simulink model "Chaotic_synchronization_Neelabhro"  (R2019a)
settings: Solver=ode45  StartTime=0.0  StopTime=100  RelTol=1e-3  EnableMultiTasking=on
settings Model: Creator=Administrator  LastModifiedBy=ar-neelabhro.roy
settings DataIOCC: LimitDataPoints=on  SaveFormat=Array  ReturnWorkspaceOutputs=off
settings OptimizationCC: LifeSpan=inf
settings DebuggingCC: SolverPrmCheckMsg=warning  AllowSymbolicDim=off  SFUnexpectedBacktrackingDiag=warning  SFNoUnconditionalDefaultTransitionDiag=warning  SFExecutionAtInitializationDiag=none  ArithmeticOperatorsInVariantConditions=warning
settings HardwareCC: ProdBitPerPointer=32  ProdBitPerSizeT=32  ProdBitPerPtrDiffT=32  ProdLargestAtomicFloat=None  ProdIntDivRoundTo=Undefined  ProdEndianess=Unspecified  ProdWordSize=32  ProdHWDeviceType=32-bit Generic
settings ModelReferenceCC: PropagateSignalLabelsOutOfModel=off
settings SFSimCC: SimUseLocalCustomCode=off
settings RTWCC: RTWUseLocalCustomCode=off
settings CodeAppCC: StateflowObjectComments=on
settings GRTTargetCC: TargetLangStandard=C89/C90 (ANSI)  GeneratePreprocessorConditionals=Disable all
settings ConfigComp: CovMetricSettings=dw  CovHtmlReporting=on  CovSaveCumulativeToWorkspaceVar=on  CovSaveSingleToWorkspaceVar=on  CovExternalEMLEnable=off  CovSFcnEnable=off

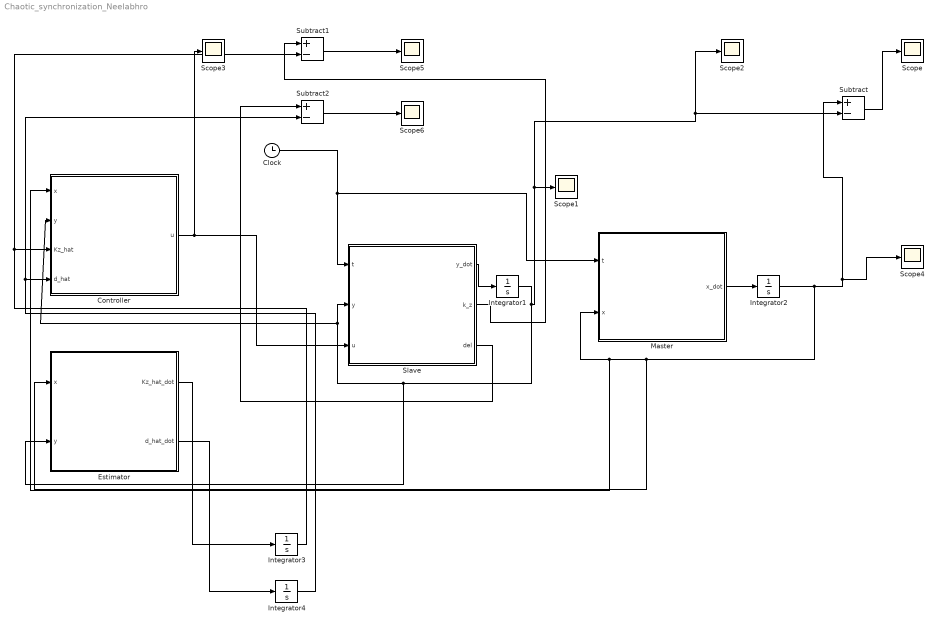
== system Chaotic_synchronization_Neelabhro ==
  Clock : Clock
      settings: Decimation=50
  Controller : MATLAB Function  TreatAsAtomicUnit=on
  Estimator : MATLAB Function  TreatAsAtomicUnit=on
  Integrator1 : Integrator  InitialCondition=[0.015; 0.001; 0.005]
  Integrator2 : Integrator  InitialCondition=[0.01; 0.002; 0.01]
  Integrator3 : Integrator  InitialCondition=[0;0;0]
  Integrator4 : Integrator  InitialCondition=[0]
  Master : MATLAB Function  TreatAsAtomicUnit=on
  Scope{,1..6} (7 alike) : Scope
  Slave : MATLAB Function  TreatAsAtomicUnit=on
  Subtract : Sum  Inputs=+-
  Subtract1 : Sum  Inputs=+-
  Subtract2 : Sum  Inputs=+-
  wires:
  Clock/1 -> Master/1(t), Slave/1(t)
  Slave/1(y_dot) -> Integrator1/1
  Master/1(x_dot) -> Integrator2/1
  Subtract/1 -> Scope/1
  Integrator2/1 -> Estimator/1(x), Controller/1(x), Master/2(x), Subtract/1, Scope4/1
  Integrator1/1 -> Estimator/2(y), Controller/2(y), Slave/2(y), Scope1/1, Scope2/1, Subtract/2
  Estimator/1(Kz_hat_dot) -> Integrator3/1
  Estimator/2(d_hat_dot) -> Integrator4/1
  Integrator3/1 -> Subtract1/2, Controller/3(Kz_hat)
  Integrator4/1 -> Subtract2/2, Controller/4(d_hat)
  Controller/1(u) -> Scope3/1, Slave/3(u)
  Slave/2(k_z) -> Subtract1/1
  Subtract1/1 -> Scope5/1
  Slave/3(del) -> Subtract2/1
  Subtract2/1 -> Scope6/1

== matlab function Chaotic_synchronization_Neelabhro/Slave ==
  data: y_dot output; t input; y input; u input; k_z output; del output
function [y_dot,k_z,del] = slave(t,y,u)

a=1.2;
b=2.92;
c=6;


am = 10;
bm = 25;
cm = 19;

kc = c - cm;
kb = b - bm;
ka = a - am;

d = 1;
k_z = [kc; kb; ka];
A = [0 1 0; 0 0 1; -c -b -a];
B = [0; 0; 1];

del = d*y(1,1)^2;
y_dot = A*y+B*(del+u);

end

== matlab function Chaotic_synchronization_Neelabhro/Controller ==
  data: x input; y input; u output; Kz_hat input; d_hat input
function u = slave(x,y,Kz_hat,d_hat)

z = y - x;
phi = y(1,1)^2 - x(1,1)^2;
u = (Kz_hat)'*z-d_hat*phi;

end

== matlab function Chaotic_synchronization_Neelabhro/Master ==
  data: t input; x_dot output; x input
function x_dot  = master(t,x)
a=1.2;
b=2.92;
c=6;
d=1;
A=[0 1 0; 0 0 1; -c -b -a];

B=[0;0;1];
del=d*x(1,1)^2;
x_dot=A*x+B*del;
end

== matlab function Chaotic_synchronization_Neelabhro/Estimator ==
  data: x input; Kz_hat_dot output; y input; d_hat_dot output
function [Kz_hat_dot, d_hat_dot]  =  Estimator(x,y)

phi = y(1,1)^2 - x(1,1)^2;
gamma = eye(3);
z = y-x;
B =[0;0;1];

P = [ 20.67, 13.54, 0.26; 13.54, 21.50, 0.74; 0.26, 0.74, 0.57];
g_d=5;

Kz_hat_dot = -gamma*z*B'*P*z;
d_hat_dot = g_d*phi*B'*P*z;


end
